simulink model "TxSteering_RxMVDR_4x4_HDL_IQ"  (R2020a)
settings: Solver=FixedStepDiscrete  StartTime=0.0  StopTime=stoptime*0 + inf  RelTol=1e-3
PreLoadFcn:
  | load('iq_bus_obj.mat');
  | model_init
InitFcn:
  | model_init
model workspace (MAT data in the model file):
  socvcb : containers.Map (value not decoded)
values from neighbouring files (symbols this model uses):
  BackSubstitutePrototype = fi(0, matrixdivbacksub_dt)    [model_init.m]
  DataSampleRate = ConverterSampleRate/DecimInterpFactor    (= 245760000)    [model_init.m]
  fc = ConverterSampleRate/4    (= 491520000)    [model_init.m]
  FPGAClkRate = DataSampleRate/VectorSamplingFactor    (= 245760000)    [model_init.m]
  matrixDivDelay = NumberOfCORDICIterations*10 + 86    [model_init.m]
  movavg_bitshift = nextpow2(sqrt(windowSize))    [model_init.m]
  mvdrPipelineDelay = covMatDelay+movAvgDelay+matrixDivDelay+normResponseDelay    [model_init.m]
  NCO_bits = 14    [model_init.m]
  numArrayElements = 4    [model_init.m]
  NumberOfCORDICIterations = matrixdivin_dt.WordLength - 1    [model_init.m]
  S2MM_frame_size = FrameSize*4    (= 40000)    [host_io_init.m]    (also in model_init.m = 1000)
  windowSize = 1024    [model_init.m]
undefined symbols (not defined in the file or in its folder): Fo, Fs, N, physconst
libraries: hdlsllib x268, simulink x53, dspsolvers x1, embreciprocals x1, dsphdlsigops x1
(part 6 of 12)

== system TxSteering_RxMVDR_4x4_HDL_IQ/DUT/MVDR/Compute Weight Vector/Matrix Left Divide/CORDIC/4x4 Complex CORDIC Matrix Left Divide/Q'B, R 4x4 Complex CORDIC Systolic Array/Leading Complex Row Rotation/Rotate first element to real - 1 ==
  x : Inport
  u : Inport  Port=2
  validIn : Inport  Port=3
  Complex to Real-Imag : ComplexToRealImag
  Complex to Real-Imag1 : ComplexToRealImag
  Delay{4..7,9..10,15} (7 alike) : Delay  DelayLength=1
  Force imaginary part to exactly zero : MATLAB Function  TreatAsAtomicUnit=on
  Inverse CORDIC Gain1 : Subsystem  TreatAsAtomicUnit=on  mask{NumberOfCORDICIterations=NumberOfCORDICIterations}
      mask prompts: NumberOfCORDICIterations "Number of CORDIC Iterations"
      mask Display: disp('1/An')
  Inverse CORDIC Gain2 : Subsystem  TreatAsAtomicUnit=on  mask{NumberOfCORDICIterations=NumberOfCORDICIterations}
      mask prompts: NumberOfCORDICIterations "Number of CORDIC Iterations"
      mask Display: disp('1/An')
  Inverse CORDIC Gain3 : Subsystem  TreatAsAtomicUnit=on  mask{NumberOfCORDICIterations=NumberOfCORDICIterations}
      mask prompts: NumberOfCORDICIterations "Number of CORDIC Iterations"
      mask Display: disp('1/An')
  Inverse CORDIC Gain4 : Subsystem  TreatAsAtomicUnit=on  mask{NumberOfCORDICIterations=NumberOfCORDICIterations}
      mask prompts: NumberOfCORDICIterations "Number of CORDIC Iterations"
      mask Display: disp('1/An')
  "Q'B, R Row Rotations - Real" : Subsystem  TreatAsAtomicUnit=on  mask{NumberOfCORDICIterations=NumberOfCORDICIterations}
      mask prompts: NumberOfCORDICIterations "Number of CORDIC Iterations"
  QR 3rd and 4th Quadrant Compensation : MATLAB Function  TreatAsAtomicUnit=on
  Real-Imag to Complex : RealImagToComplex
  Real-Imag to Complex1 : RealImagToComplex
  State Control : StateControl  StateControl=Synchronous
  Unit Delay Enabled Synchronous{,1..3} (4 alike) : hdlsllib/Discrete/Unit Delay Enabled Synchronous  InitialCondition=0.0  SampleTime=-1
      settings: SourceProductBaseCode=SL
  ValidIn to Ready Logic with Delay : Subsystem
  x' : Outport  VectorParamsAs1DForOutWhenUnconnected=off
  u' : Outport  Port=2  VectorParamsAs1DForOutWhenUnconnected=off
  validOut : Outport  Port=3  VectorParamsAs1DForOutWhenUnconnected=off
  ready : Outport  Port=4  VectorParamsAs1DForOutWhenUnconnected=off
  wires:
  Unit Delay Enabled Synchronous3/1 -> x'/1
  Real-Imag to Complex/1 -> Unit Delay Enabled Synchronous3/1
  Unit Delay Enabled Synchronous2/1 -> u'/1
  Real-Imag to Complex1/1 -> Unit Delay Enabled Synchronous2/1
  Unit Delay Enabled Synchronous1/1 -> Complex to Real-Imag/1
  Unit Delay Enabled Synchronous/1 -> Complex to Real-Imag1/1
  "Q'B, R Row Rotations - Real"/6(ready) -> ValidIn to Ready Logic with Delay/1(readyIn)
  ValidIn to Ready Logic with Delay/1(readyOut) -> ready/1
  Delay15/1 -> validOut/1
  "Q'B, R Row Rotations - Real"/5(validOut) -> Delay15/1, Unit Delay Enabled Synchronous3/2, Unit Delay Enabled Synchronous2/2
  Inverse CORDIC Gain3/1(Out1) -> Real-Imag to Complex1/2
  Inverse CORDIC Gain2/1(Out1) -> Real-Imag to Complex1/1
  Inverse CORDIC Gain1/1(Out1) -> Force imaginary part to exactly zero/1(u)
  Inverse CORDIC Gain4/1(Out1) -> Real-Imag to Complex/1
  Delay10/1 -> "Q'B, R Row Rotations - Real"/5(validIn), ValidIn to Ready Logic with Delay/2(validIn * z^-1)
  validIn/1 -> Delay9/1, Unit Delay Enabled Synchronous1/2, Unit Delay Enabled Synchronous/2
  Delay9/1 -> Delay10/1, ValidIn to Ready Logic with Delay/3(validIn)
  Force imaginary part to exactly zero/1(y) -> Real-Imag to Complex/2
  "Q'B, R Row Rotations - Real"/2(y_out) -> Inverse CORDIC Gain1/1(In1)
  u/1 -> Unit Delay Enabled Synchronous/1
  x/1 -> Unit Delay Enabled Synchronous1/1
  "Q'B, R Row Rotations - Real"/4(v_out) -> Inverse CORDIC Gain3/1(In1)
  "Q'B, R Row Rotations - Real"/3(u_out) -> Inverse CORDIC Gain2/1(In1)
  "Q'B, R Row Rotations - Real"/1(x_out) -> Inverse CORDIC Gain4/1(In1)
  Delay7/1 -> "Q'B, R Row Rotations - Real"/4(v)
  Delay6/1 -> "Q'B, R Row Rotations - Real"/3(u)
  Delay5/1 -> "Q'B, R Row Rotations - Real"/2(y)
  Delay4/1 -> "Q'B, R Row Rotations - Real"/1(x)
  Complex to Real-Imag1/2 -> QR 3rd and 4th Quadrant Compensation/4(v)
  Complex to Real-Imag1/1 -> QR 3rd and 4th Quadrant Compensation/3(u)
  Complex to Real-Imag/2 -> QR 3rd and 4th Quadrant Compensation/2(y)
  Complex to Real-Imag/1 -> QR 3rd and 4th Quadrant Compensation/1(x)
  QR 3rd and 4th Quadrant Compensation/4(v_out) -> Delay7/1
  QR 3rd and 4th Quadrant Compensation/2(y_out) -> Delay5/1
  QR 3rd and 4th Quadrant Compensation/3(u_out) -> Delay6/1
  QR 3rd and 4th Quadrant Compensation/1(x_out) -> Delay4/1

== system TxSteering_RxMVDR_4x4_HDL_IQ/DUT/MVDR/Compute Weight Vector/Matrix Left Divide/CORDIC/4x4 Complex CORDIC Matrix Left Divide/Q'B, R 4x4 Complex CORDIC Systolic Array/Leading Complex Row Rotation/ValidIn to Ready Logic ==
  readyIn : Inport
  validIn : Inport  Port=2
  AND : Logic  IconShape=distinctive  AllPortsSameDT=off  OutDataTypeStr=boolean
  NOT : Logic  Operator=NOT  IconShape=distinctive  AllPortsSameDT=off  OutDataTypeStr=boolean
  readyOut : Outport  VectorParamsAs1DForOutWhenUnconnected=off
  wires:
  validIn/1 -> NOT/1
  readyIn/1 -> AND/1
  AND/1 -> readyOut/1
  NOT/1 -> AND/2

== system TxSteering_RxMVDR_4x4_HDL_IQ/DUT/MVDR/Compute Weight Vector/Matrix Left Divide/CORDIC/4x4 Complex CORDIC Matrix Left Divide/Q'B, R 4x4 Complex CORDIC Systolic Array/Leading Complex Row Rotation/ValidIn to Ready Logic1 ==
  readyIn : Inport
  validIn : Inport  Port=2
  AND : Logic  IconShape=distinctive  AllPortsSameDT=off  OutDataTypeStr=boolean
  NOT : Logic  Operator=NOT  IconShape=distinctive  AllPortsSameDT=off  OutDataTypeStr=boolean
  readyOut : Outport  VectorParamsAs1DForOutWhenUnconnected=off
  wires:
  validIn/1 -> NOT/1
  readyIn/1 -> AND/1
  AND/1 -> readyOut/1
  NOT/1 -> AND/2

== system TxSteering_RxMVDR_4x4_HDL_IQ/DUT/MVDR/Compute Weight Vector/Matrix Left Divide/CORDIC/4x4 Complex CORDIC Matrix Left Divide/Q'B, R 4x4 Complex CORDIC Systolic Array/Leading Complex Row Rotation - 2/Inverse CORDIC Gain1 ==
  In1 : Inport
  Inverse CORDIC Gain : Gain  Gain=1/prod(sqrt(1+2.^(-2*(0:double(NumberOfCORDICIterations)-1))))  OutDataTypeStr=Inherit: Same as input
  Out1 : Outport  VectorParamsAs1DForOutWhenUnconnected=off
  wires:
  Inverse CORDIC Gain/1 -> Out1/1
  In1/1 -> Inverse CORDIC Gain/1

== system TxSteering_RxMVDR_4x4_HDL_IQ/DUT/MVDR/Compute Weight Vector/Matrix Left Divide/CORDIC/4x4 Complex CORDIC Matrix Left Divide/Q'B, R 4x4 Complex CORDIC Systolic Array/Leading Complex Row Rotation - 2/Inverse CORDIC Gain2 ==
  In1 : Inport
  Inverse CORDIC Gain : Gain  Gain=1/prod(sqrt(1+2.^(-2*(0:double(NumberOfCORDICIterations)-1))))  OutDataTypeStr=Inherit: Same as input
  Out1 : Outport  VectorParamsAs1DForOutWhenUnconnected=off
  wires:
  Inverse CORDIC Gain/1 -> Out1/1
  In1/1 -> Inverse CORDIC Gain/1

== system TxSteering_RxMVDR_4x4_HDL_IQ/DUT/MVDR/Compute Weight Vector/Matrix Left Divide/CORDIC/4x4 Complex CORDIC Matrix Left Divide/Q'B, R 4x4 Complex CORDIC Systolic Array/Leading Complex Row Rotation - 2/Inverse CORDIC Gain3 ==
  In1 : Inport
  Inverse CORDIC Gain : Gain  Gain=1/prod(sqrt(1+2.^(-2*(0:double(NumberOfCORDICIterations)-1))))  OutDataTypeStr=Inherit: Same as input
  Out1 : Outport  VectorParamsAs1DForOutWhenUnconnected=off
  wires:
  Inverse CORDIC Gain/1 -> Out1/1
  In1/1 -> Inverse CORDIC Gain/1

== system TxSteering_RxMVDR_4x4_HDL_IQ/DUT/MVDR/Compute Weight Vector/Matrix Left Divide/CORDIC/4x4 Complex CORDIC Matrix Left Divide/Q'B, R 4x4 Complex CORDIC Systolic Array/Leading Complex Row Rotation - 2/Inverse CORDIC Gain4 ==
  In1 : Inport
  Inverse CORDIC Gain : Gain  Gain=1/prod(sqrt(1+2.^(-2*(0:double(NumberOfCORDICIterations)-1))))  OutDataTypeStr=Inherit: Same as input
  Out1 : Outport  VectorParamsAs1DForOutWhenUnconnected=off
  wires:
  Inverse CORDIC Gain/1 -> Out1/1
  In1/1 -> Inverse CORDIC Gain/1

== system TxSteering_RxMVDR_4x4_HDL_IQ/DUT/MVDR/Compute Weight Vector/Matrix Left Divide/CORDIC/4x4 Complex CORDIC Matrix Left Divide/Q'B, R 4x4 Complex CORDIC Systolic Array/Leading Complex Row Rotation - 2/Q'B, R Row Rotations - Complex ==
  x : Inport
  y : Inport  Port=2
  u : Inport  Port=3
  v : Inport  Port=4
  validIn : Inport  Port=5
  CORDIC Counter : Subsystem  mask{NumberOfCORDICIterations=NumberOfCORDICIterations}
      mask prompts: NumberOfCORDICIterations "Number of CORDIC Iterations"
  Delay{1..13} (13 alike) : Delay  DelayLength=1
  MATLAB Function : MATLAB Function  TreatAsAtomicUnit=on
  Same Datatype : Subsystem  TreatAsAtomicUnit=on
  Same Datatype1 : Subsystem  TreatAsAtomicUnit=on
  Same Datatype2 : Subsystem  TreatAsAtomicUnit=on
  Same Datatype3 : Subsystem  TreatAsAtomicUnit=on
  Switch{,1..3} (4 alike) : Switch  Criteria=u2 ~= 0
  x_out : Outport  VectorParamsAs1DForOutWhenUnconnected=off
  y_out : Outport  Port=2  VectorParamsAs1DForOutWhenUnconnected=off
  u_out : Outport  Port=3  VectorParamsAs1DForOutWhenUnconnected=off
  v_out : Outport  Port=4  VectorParamsAs1DForOutWhenUnconnected=off
  validOut : Outport  Port=5  VectorParamsAs1DForOutWhenUnconnected=off
  ready : Outport  Port=6  VectorParamsAs1DForOutWhenUnconnected=off
  wires:
  Delay1/1 -> Same Datatype/1(Data), x_out/1
  Delay2/1 -> Same Datatype1/1(Data), y_out/1
  Delay11/1 -> Same Datatype2/1(Data), v_out/1
  MATLAB Function/1(x_out) -> Delay1/1
  MATLAB Function/2(y_out) -> Delay2/1
  MATLAB Function/3(u_out) -> Delay7/1
  MATLAB Function/4(v_out) -> Delay11/1
  Delay7/1 -> Same Datatype3/1(Data), u_out/1
  Delay3/1 -> validOut/1
  validIn/1 -> CORDIC Counter/1(validIn)
  CORDIC Counter/2(count) -> Delay10/1
  CORDIC Counter/3(last) -> Delay12/1
  CORDIC Counter/4(ready) -> Delay13/1
  Switch/1 -> MATLAB Function/1(x)
  Switch1/1 -> MATLAB Function/2(y)
  Switch2/1 -> MATLAB Function/3(u)
  Switch3/1 -> MATLAB Function/4(v)
  CORDIC Counter/1(count_is_positive) -> Delay9/1
  x/1 -> Delay4/1
  y/1 -> Delay5/1
  u/1 -> Delay6/1
  v/1 -> Delay8/1
  Same Datatype/1(DataOut) -> Switch/1
  Same Datatype1/1(DataOut) -> Switch1/1
  Same Datatype3/1(DataOut) -> Switch2/1
  Same Datatype2/1(DataOut) -> Switch3/1
  Delay4/1 -> Same Datatype/2(Reference), Switch/3
  Delay5/1 -> Same Datatype1/2(Reference), Switch1/3
  Delay6/1 -> Same Datatype3/2(Reference), Switch2/3
  Delay8/1 -> Same Datatype2/2(Reference), Switch3/3
  Delay9/1 -> Switch/2, Switch1/2, Switch2/2, Switch3/2
  Delay10/1 -> MATLAB Function/5(iteration)
  Delay12/1 -> Delay3/1
  Delay13/1 -> ready/1

== system TxSteering_RxMVDR_4x4_HDL_IQ/DUT/MVDR/Compute Weight Vector/Matrix Left Divide/CORDIC/4x4 Complex CORDIC Matrix Left Divide/Q'B, R 4x4 Complex CORDIC Systolic Array/Leading Complex Row Rotation - 2/Rotate first element to real ==
  x : Inport
  u : Inport  Port=2
  validIn : Inport  Port=3
  Complex to Real-Imag : ComplexToRealImag
  Complex to Real-Imag1 : ComplexToRealImag
  Delay{4..7,9..10,15} (7 alike) : Delay  DelayLength=1
  Force imaginary part to exactly zero : MATLAB Function  TreatAsAtomicUnit=on
  Inverse CORDIC Gain1 : Subsystem  TreatAsAtomicUnit=on  mask{NumberOfCORDICIterations=NumberOfCORDICIterations}
      mask prompts: NumberOfCORDICIterations "Number of CORDIC Iterations"
      mask Display: disp('1/An')
  Inverse CORDIC Gain2 : Subsystem  TreatAsAtomicUnit=on  mask{NumberOfCORDICIterations=NumberOfCORDICIterations}
      mask prompts: NumberOfCORDICIterations "Number of CORDIC Iterations"
      mask Display: disp('1/An')
  Inverse CORDIC Gain3 : Subsystem  TreatAsAtomicUnit=on  mask{NumberOfCORDICIterations=NumberOfCORDICIterations}
      mask prompts: NumberOfCORDICIterations "Number of CORDIC Iterations"
      mask Display: disp('1/An')
  Inverse CORDIC Gain4 : Subsystem  TreatAsAtomicUnit=on  mask{NumberOfCORDICIterations=NumberOfCORDICIterations}
      mask prompts: NumberOfCORDICIterations "Number of CORDIC Iterations"
      mask Display: disp('1/An')
  "Q'B, R Row Rotations - Real" : Subsystem  TreatAsAtomicUnit=on  mask{NumberOfCORDICIterations=NumberOfCORDICIterations}
      mask prompts: NumberOfCORDICIterations "Number of CORDIC Iterations"
  QR 3rd and 4th Quadrant Compensation : MATLAB Function  TreatAsAtomicUnit=on
  Real-Imag to Complex : RealImagToComplex
  Real-Imag to Complex1 : RealImagToComplex
  State Control : StateControl  StateControl=Synchronous
  Unit Delay Enabled Synchronous{,1..3} (4 alike) : hdlsllib/Discrete/Unit Delay Enabled Synchronous  InitialCondition=0.0  SampleTime=-1
      settings: SourceProductBaseCode=SL
  ValidIn to Ready Logic with Delay : Subsystem
  x' : Outport  VectorParamsAs1DForOutWhenUnconnected=off
  u' : Outport  Port=2  VectorParamsAs1DForOutWhenUnconnected=off
  validOut : Outport  Port=3  VectorParamsAs1DForOutWhenUnconnected=off
  ready : Outport  Port=4  VectorParamsAs1DForOutWhenUnconnected=off
  wires:
  Unit Delay Enabled Synchronous3/1 -> x'/1
  Real-Imag to Complex/1 -> Unit Delay Enabled Synchronous3/1
  Unit Delay Enabled Synchronous2/1 -> u'/1
  Real-Imag to Complex1/1 -> Unit Delay Enabled Synchronous2/1
  Unit Delay Enabled Synchronous1/1 -> Complex to Real-Imag/1
  Unit Delay Enabled Synchronous/1 -> Complex to Real-Imag1/1
  "Q'B, R Row Rotations - Real"/6(ready) -> ValidIn to Ready Logic with Delay/1(readyIn)
  ValidIn to Ready Logic with Delay/1(readyOut) -> ready/1
  Delay15/1 -> validOut/1
  "Q'B, R Row Rotations - Real"/5(validOut) -> Delay15/1, Unit Delay Enabled Synchronous3/2, Unit Delay Enabled Synchronous2/2
  Inverse CORDIC Gain3/1(Out1) -> Real-Imag to Complex1/2
  Inverse CORDIC Gain2/1(Out1) -> Real-Imag to Complex1/1
  Inverse CORDIC Gain1/1(Out1) -> Force imaginary part to exactly zero/1(u)
  Inverse CORDIC Gain4/1(Out1) -> Real-Imag to Complex/1
  Delay10/1 -> "Q'B, R Row Rotations - Real"/5(validIn), ValidIn to Ready Logic with Delay/2(validIn * z^-1)
  validIn/1 -> Delay9/1, Unit Delay Enabled Synchronous1/2, Unit Delay Enabled Synchronous/2
  Delay9/1 -> Delay10/1, ValidIn to Ready Logic with Delay/3(validIn)
  Force imaginary part to exactly zero/1(y) -> Real-Imag to Complex/2
  "Q'B, R Row Rotations - Real"/2(y_out) -> Inverse CORDIC Gain1/1(In1)
  u/1 -> Unit Delay Enabled Synchronous/1
  x/1 -> Unit Delay Enabled Synchronous1/1
  "Q'B, R Row Rotations - Real"/4(v_out) -> Inverse CORDIC Gain3/1(In1)
  "Q'B, R Row Rotations - Real"/3(u_out) -> Inverse CORDIC Gain2/1(In1)
  "Q'B, R Row Rotations - Real"/1(x_out) -> Inverse CORDIC Gain4/1(In1)
  Delay7/1 -> "Q'B, R Row Rotations - Real"/4(v)
  Delay6/1 -> "Q'B, R Row Rotations - Real"/3(u)
  Delay5/1 -> "Q'B, R Row Rotations - Real"/2(y)
  Delay4/1 -> "Q'B, R Row Rotations - Real"/1(x)
  Complex to Real-Imag1/2 -> QR 3rd and 4th Quadrant Compensation/4(v)
  Complex to Real-Imag1/1 -> QR 3rd and 4th Quadrant Compensation/3(u)
  Complex to Real-Imag/2 -> QR 3rd and 4th Quadrant Compensation/2(y)
  Complex to Real-Imag/1 -> QR 3rd and 4th Quadrant Compensation/1(x)
  QR 3rd and 4th Quadrant Compensation/4(v_out) -> Delay7/1
  QR 3rd and 4th Quadrant Compensation/2(y_out) -> Delay5/1
  QR 3rd and 4th Quadrant Compensation/3(u_out) -> Delay6/1
  QR 3rd and 4th Quadrant Compensation/1(x_out) -> Delay4/1

== system TxSteering_RxMVDR_4x4_HDL_IQ/DUT/MVDR/Compute Weight Vector/Matrix Left Divide/CORDIC/4x4 Complex CORDIC Matrix Left Divide/Q'B, R 4x4 Complex CORDIC Systolic Array/Leading Complex Row Rotation - 2/Rotate first element to real - 1 ==
  x : Inport
  u : Inport  Port=2
  validIn : Inport  Port=3
  Complex to Real-Imag : ComplexToRealImag
  Complex to Real-Imag1 : ComplexToRealImag
  Delay{4..7,9..10,15} (7 alike) : Delay  DelayLength=1
  Force imaginary part to exactly zero : MATLAB Function  TreatAsAtomicUnit=on
  Inverse CORDIC Gain1 : Subsystem  TreatAsAtomicUnit=on  mask{NumberOfCORDICIterations=NumberOfCORDICIterations}
      mask prompts: NumberOfCORDICIterations "Number of CORDIC Iterations"
      mask Display: disp('1/An')
  Inverse CORDIC Gain2 : Subsystem  TreatAsAtomicUnit=on  mask{NumberOfCORDICIterations=NumberOfCORDICIterations}
      mask prompts: NumberOfCORDICIterations "Number of CORDIC Iterations"
      mask Display: disp('1/An')
  Inverse CORDIC Gain3 : Subsystem  TreatAsAtomicUnit=on  mask{NumberOfCORDICIterations=NumberOfCORDICIterations}
      mask prompts: NumberOfCORDICIterations "Number of CORDIC Iterations"
      mask Display: disp('1/An')
  Inverse CORDIC Gain4 : Subsystem  TreatAsAtomicUnit=on  mask{NumberOfCORDICIterations=NumberOfCORDICIterations}
      mask prompts: NumberOfCORDICIterations "Number of CORDIC Iterations"
      mask Display: disp('1/An')
  "Q'B, R Row Rotations - Real" : Subsystem  TreatAsAtomicUnit=on  mask{NumberOfCORDICIterations=NumberOfCORDICIterations}
      mask prompts: NumberOfCORDICIterations "Number of CORDIC Iterations"
  QR 3rd and 4th Quadrant Compensation : MATLAB Function  TreatAsAtomicUnit=on
  Real-Imag to Complex : RealImagToComplex
  Real-Imag to Complex1 : RealImagToComplex
  State Control : StateControl  StateControl=Synchronous
  Unit Delay Enabled Synchronous{,1..3} (4 alike) : hdlsllib/Discrete/Unit Delay Enabled Synchronous  InitialCondition=0.0  SampleTime=-1
      settings: SourceProductBaseCode=SL
  ValidIn to Ready Logic with Delay : Subsystem
  x' : Outport  VectorParamsAs1DForOutWhenUnconnected=off
  u' : Outport  Port=2  VectorParamsAs1DForOutWhenUnconnected=off
  validOut : Outport  Port=3  VectorParamsAs1DForOutWhenUnconnected=off
  ready : Outport  Port=4  VectorParamsAs1DForOutWhenUnconnected=off
  wires:
  QR 3rd and 4th Quadrant Compensation/1(x_out) -> Delay4/1
  QR 3rd and 4th Quadrant Compensation/3(u_out) -> Delay6/1
  QR 3rd and 4th Quadrant Compensation/2(y_out) -> Delay5/1
  QR 3rd and 4th Quadrant Compensation/4(v_out) -> Delay7/1
  Complex to Real-Imag/1 -> QR 3rd and 4th Quadrant Compensation/1(x)
  Complex to Real-Imag/2 -> QR 3rd and 4th Quadrant Compensation/2(y)
  Complex to Real-Imag1/1 -> QR 3rd and 4th Quadrant Compensation/3(u)
  Complex to Real-Imag1/2 -> QR 3rd and 4th Quadrant Compensation/4(v)
  Delay4/1 -> "Q'B, R Row Rotations - Real"/1(x)
  Delay5/1 -> "Q'B, R Row Rotations - Real"/2(y)
  Delay6/1 -> "Q'B, R Row Rotations - Real"/3(u)
  Delay7/1 -> "Q'B, R Row Rotations - Real"/4(v)
  "Q'B, R Row Rotations - Real"/1(x_out) -> Inverse CORDIC Gain4/1(In1)
  "Q'B, R Row Rotations - Real"/3(u_out) -> Inverse CORDIC Gain2/1(In1)
  "Q'B, R Row Rotations - Real"/4(v_out) -> Inverse CORDIC Gain3/1(In1)
  x/1 -> Unit Delay Enabled Synchronous1/1
  u/1 -> Unit Delay Enabled Synchronous/1
  "Q'B, R Row Rotations - Real"/2(y_out) -> Inverse CORDIC Gain1/1(In1)
  Force imaginary part to exactly zero/1(y) -> Real-Imag to Complex/2
  Delay9/1 -> ValidIn to Ready Logic with Delay/3(validIn), Delay10/1
  validIn/1 -> Unit Delay Enabled Synchronous/2, Unit Delay Enabled Synchronous1/2, Delay9/1
  Delay10/1 -> ValidIn to Ready Logic with Delay/2(validIn * z^-1), "Q'B, R Row Rotations - Real"/5(validIn)
  Inverse CORDIC Gain4/1(Out1) -> Real-Imag to Complex/1
  Inverse CORDIC Gain1/1(Out1) -> Force imaginary part to exactly zero/1(u)
  Inverse CORDIC Gain2/1(Out1) -> Real-Imag to Complex1/1
  Inverse CORDIC Gain3/1(Out1) -> Real-Imag to Complex1/2
  "Q'B, R Row Rotations - Real"/5(validOut) -> Unit Delay Enabled Synchronous2/2, Unit Delay Enabled Synchronous3/2, Delay15/1
  Delay15/1 -> validOut/1
  ValidIn to Ready Logic with Delay/1(readyOut) -> ready/1
  "Q'B, R Row Rotations - Real"/6(ready) -> ValidIn to Ready Logic with Delay/1(readyIn)
  Unit Delay Enabled Synchronous/1 -> Complex to Real-Imag1/1
  Unit Delay Enabled Synchronous1/1 -> Complex to Real-Imag/1
  Real-Imag to Complex1/1 -> Unit Delay Enabled Synchronous2/1
  Unit Delay Enabled Synchronous2/1 -> u'/1
  Real-Imag to Complex/1 -> Unit Delay Enabled Synchronous3/1
  Unit Delay Enabled Synchronous3/1 -> x'/1

== system TxSteering_RxMVDR_4x4_HDL_IQ/DUT/MVDR/Compute Weight Vector/Matrix Left Divide/CORDIC/4x4 Complex CORDIC Matrix Left Divide/Q'B, R 4x4 Complex CORDIC Systolic Array/Leading Complex Row Rotation - 2/ValidIn to Ready Logic ==
  readyIn : Inport
  validIn : Inport  Port=2
  AND : Logic  IconShape=distinctive  AllPortsSameDT=off  OutDataTypeStr=boolean
  NOT : Logic  Operator=NOT  IconShape=distinctive  AllPortsSameDT=off  OutDataTypeStr=boolean
  readyOut : Outport  VectorParamsAs1DForOutWhenUnconnected=off
  wires:
  validIn/1 -> NOT/1
  readyIn/1 -> AND/1
  AND/1 -> readyOut/1
  NOT/1 -> AND/2

== system TxSteering_RxMVDR_4x4_HDL_IQ/DUT/MVDR/Compute Weight Vector/Matrix Left Divide/CORDIC/4x4 Complex CORDIC Matrix Left Divide/Q'B, R 4x4 Complex CORDIC Systolic Array/Leading Complex Row Rotation - 2/ValidIn to Ready Logic1 ==
  readyIn : Inport
  validIn : Inport  Port=2
  AND : Logic  IconShape=distinctive  AllPortsSameDT=off  OutDataTypeStr=boolean
  NOT : Logic  Operator=NOT  IconShape=distinctive  AllPortsSameDT=off  OutDataTypeStr=boolean
  readyOut : Outport  VectorParamsAs1DForOutWhenUnconnected=off
  wires:
  validIn/1 -> NOT/1
  readyIn/1 -> AND/1
  AND/1 -> readyOut/1
  NOT/1 -> AND/2

== system TxSteering_RxMVDR_4x4_HDL_IQ/DUT/MVDR/Compute Weight Vector/Matrix Left Divide/CORDIC/4x4 Complex CORDIC Matrix Left Divide/Q'B, R 4x4 Complex CORDIC Systolic Array/Leading Complex Row Rotation - 3/Inverse CORDIC Gain1 ==
  In1 : Inport
  Inverse CORDIC Gain : Gain  Gain=1/prod(sqrt(1+2.^(-2*(0:double(NumberOfCORDICIterations)-1))))  OutDataTypeStr=Inherit: Same as input
  Out1 : Outport  VectorParamsAs1DForOutWhenUnconnected=off
  wires:
  Inverse CORDIC Gain/1 -> Out1/1
  In1/1 -> Inverse CORDIC Gain/1

== system TxSteering_RxMVDR_4x4_HDL_IQ/DUT/MVDR/Compute Weight Vector/Matrix Left Divide/CORDIC/4x4 Complex CORDIC Matrix Left Divide/Q'B, R 4x4 Complex CORDIC Systolic Array/Leading Complex Row Rotation - 3/Inverse CORDIC Gain2 ==
  In1 : Inport
  Inverse CORDIC Gain : Gain  Gain=1/prod(sqrt(1+2.^(-2*(0:double(NumberOfCORDICIterations)-1))))  OutDataTypeStr=Inherit: Same as input
  Out1 : Outport  VectorParamsAs1DForOutWhenUnconnected=off
  wires:
  Inverse CORDIC Gain/1 -> Out1/1
  In1/1 -> Inverse CORDIC Gain/1

== system TxSteering_RxMVDR_4x4_HDL_IQ/DUT/MVDR/Compute Weight Vector/Matrix Left Divide/CORDIC/4x4 Complex CORDIC Matrix Left Divide/Q'B, R 4x4 Complex CORDIC Systolic Array/Leading Complex Row Rotation - 3/Inverse CORDIC Gain3 ==
  In1 : Inport
  Inverse CORDIC Gain : Gain  Gain=1/prod(sqrt(1+2.^(-2*(0:double(NumberOfCORDICIterations)-1))))  OutDataTypeStr=Inherit: Same as input
  Out1 : Outport  VectorParamsAs1DForOutWhenUnconnected=off
  wires:
  Inverse CORDIC Gain/1 -> Out1/1
  In1/1 -> Inverse CORDIC Gain/1

== system TxSteering_RxMVDR_4x4_HDL_IQ/DUT/MVDR/Compute Weight Vector/Matrix Left Divide/CORDIC/4x4 Complex CORDIC Matrix Left Divide/Q'B, R 4x4 Complex CORDIC Systolic Array/Leading Complex Row Rotation - 3/Inverse CORDIC Gain4 ==
  In1 : Inport
  Inverse CORDIC Gain : Gain  Gain=1/prod(sqrt(1+2.^(-2*(0:double(NumberOfCORDICIterations)-1))))  OutDataTypeStr=Inherit: Same as input
  Out1 : Outport  VectorParamsAs1DForOutWhenUnconnected=off
  wires:
  Inverse CORDIC Gain/1 -> Out1/1
  In1/1 -> Inverse CORDIC Gain/1

== system TxSteering_RxMVDR_4x4_HDL_IQ/DUT/MVDR/Compute Weight Vector/Matrix Left Divide/CORDIC/4x4 Complex CORDIC Matrix Left Divide/Q'B, R 4x4 Complex CORDIC Systolic Array/Leading Complex Row Rotation - 3/Q'B, R Row Rotations - Complex ==
  x : Inport
  y : Inport  Port=2
  u : Inport  Port=3
  v : Inport  Port=4
  validIn : Inport  Port=5
  CORDIC Counter : Subsystem  mask{NumberOfCORDICIterations=NumberOfCORDICIterations}
      mask prompts: NumberOfCORDICIterations "Number of CORDIC Iterations"
  Delay{1..13} (13 alike) : Delay  DelayLength=1
  MATLAB Function : MATLAB Function  TreatAsAtomicUnit=on
  Same Datatype : Subsystem  TreatAsAtomicUnit=on
  Same Datatype1 : Subsystem  TreatAsAtomicUnit=on
  Same Datatype2 : Subsystem  TreatAsAtomicUnit=on
  Same Datatype3 : Subsystem  TreatAsAtomicUnit=on
  Switch{,1..3} (4 alike) : Switch  Criteria=u2 ~= 0
  x_out : Outport  VectorParamsAs1DForOutWhenUnconnected=off
  y_out : Outport  Port=2  VectorParamsAs1DForOutWhenUnconnected=off
  u_out : Outport  Port=3  VectorParamsAs1DForOutWhenUnconnected=off
  v_out : Outport  Port=4  VectorParamsAs1DForOutWhenUnconnected=off
  validOut : Outport  Port=5  VectorParamsAs1DForOutWhenUnconnected=off
  ready : Outport  Port=6  VectorParamsAs1DForOutWhenUnconnected=off
  wires:
  Delay13/1 -> ready/1
  Delay12/1 -> Delay3/1
  Delay10/1 -> MATLAB Function/5(iteration)
  Delay9/1 -> Switch3/2, Switch2/2, Switch1/2, Switch/2
  Delay8/1 -> Switch3/3, Same Datatype2/2(Reference)
  Delay6/1 -> Switch2/3, Same Datatype3/2(Reference)
  Delay5/1 -> Switch1/3, Same Datatype1/2(Reference)
  Delay4/1 -> Switch/3, Same Datatype/2(Reference)
  Same Datatype2/1(DataOut) -> Switch3/1
  Same Datatype3/1(DataOut) -> Switch2/1
  Same Datatype1/1(DataOut) -> Switch1/1
  Same Datatype/1(DataOut) -> Switch/1
  v/1 -> Delay8/1
  u/1 -> Delay6/1
  y/1 -> Delay5/1
  x/1 -> Delay4/1
  CORDIC Counter/1(count_is_positive) -> Delay9/1
  Switch3/1 -> MATLAB Function/4(v)
  Switch2/1 -> MATLAB Function/3(u)
  Switch1/1 -> MATLAB Function/2(y)
  Switch/1 -> MATLAB Function/1(x)
  CORDIC Counter/4(ready) -> Delay13/1
  CORDIC Counter/3(last) -> Delay12/1
  CORDIC Counter/2(count) -> Delay10/1
  validIn/1 -> CORDIC Counter/1(validIn)
  Delay3/1 -> validOut/1
  Delay7/1 -> u_out/1, Same Datatype3/1(Data)
  MATLAB Function/4(v_out) -> Delay11/1
  MATLAB Function/3(u_out) -> Delay7/1
  MATLAB Function/2(y_out) -> Delay2/1
  MATLAB Function/1(x_out) -> Delay1/1
  Delay11/1 -> v_out/1, Same Datatype2/1(Data)
  Delay2/1 -> y_out/1, Same Datatype1/1(Data)
  Delay1/1 -> x_out/1, Same Datatype/1(Data)

== system TxSteering_RxMVDR_4x4_HDL_IQ/DUT/MVDR/Compute Weight Vector/Matrix Left Divide/CORDIC/4x4 Complex CORDIC Matrix Left Divide/Q'B, R 4x4 Complex CORDIC Systolic Array/Leading Complex Row Rotation - 3/Rotate first element to real ==
  x : Inport
  u : Inport  Port=2
  validIn : Inport  Port=3
  Complex to Real-Imag : ComplexToRealImag
  Complex to Real-Imag1 : ComplexToRealImag
  Delay{4..7,9..10,15} (7 alike) : Delay  DelayLength=1
  Force imaginary part to exactly zero : MATLAB Function  TreatAsAtomicUnit=on
  Inverse CORDIC Gain1 : Subsystem  TreatAsAtomicUnit=on  mask{NumberOfCORDICIterations=NumberOfCORDICIterations}
      mask prompts: NumberOfCORDICIterations "Number of CORDIC Iterations"
      mask Display: disp('1/An')
  Inverse CORDIC Gain2 : Subsystem  TreatAsAtomicUnit=on  mask{NumberOfCORDICIterations=NumberOfCORDICIterations}
      mask prompts: NumberOfCORDICIterations "Number of CORDIC Iterations"
      mask Display: disp('1/An')
  Inverse CORDIC Gain3 : Subsystem  TreatAsAtomicUnit=on  mask{NumberOfCORDICIterations=NumberOfCORDICIterations}
      mask prompts: NumberOfCORDICIterations "Number of CORDIC Iterations"
      mask Display: disp('1/An')
  Inverse CORDIC Gain4 : Subsystem  TreatAsAtomicUnit=on  mask{NumberOfCORDICIterations=NumberOfCORDICIterations}
      mask prompts: NumberOfCORDICIterations "Number of CORDIC Iterations"
      mask Display: disp('1/An')
  "Q'B, R Row Rotations - Real" : Subsystem  TreatAsAtomicUnit=on  mask{NumberOfCORDICIterations=NumberOfCORDICIterations}
      mask prompts: NumberOfCORDICIterations "Number of CORDIC Iterations"
  QR 3rd and 4th Quadrant Compensation : MATLAB Function  TreatAsAtomicUnit=on
  Real-Imag to Complex : RealImagToComplex
  Real-Imag to Complex1 : RealImagToComplex
  State Control : StateControl  StateControl=Synchronous
  Unit Delay Enabled Synchronous{,1..3} (4 alike) : hdlsllib/Discrete/Unit Delay Enabled Synchronous  InitialCondition=0.0  SampleTime=-1
      settings: SourceProductBaseCode=SL
  ValidIn to Ready Logic with Delay : Subsystem
  x' : Outport  VectorParamsAs1DForOutWhenUnconnected=off
  u' : Outport  Port=2  VectorParamsAs1DForOutWhenUnconnected=off
  validOut : Outport  Port=3  VectorParamsAs1DForOutWhenUnconnected=off
  ready : Outport  Port=4  VectorParamsAs1DForOutWhenUnconnected=off
  wires:
  Unit Delay Enabled Synchronous3/1 -> x'/1
  Real-Imag to Complex/1 -> Unit Delay Enabled Synchronous3/1
  Unit Delay Enabled Synchronous2/1 -> u'/1
  Real-Imag to Complex1/1 -> Unit Delay Enabled Synchronous2/1
  Unit Delay Enabled Synchronous1/1 -> Complex to Real-Imag/1
  Unit Delay Enabled Synchronous/1 -> Complex to Real-Imag1/1
  "Q'B, R Row Rotations - Real"/6(ready) -> ValidIn to Ready Logic with Delay/1(readyIn)
  ValidIn to Ready Logic with Delay/1(readyOut) -> ready/1
  Delay15/1 -> validOut/1
  "Q'B, R Row Rotations - Real"/5(validOut) -> Delay15/1, Unit Delay Enabled Synchronous3/2, Unit Delay Enabled Synchronous2/2
  Inverse CORDIC Gain3/1(Out1) -> Real-Imag to Complex1/2
  Inverse CORDIC Gain2/1(Out1) -> Real-Imag to Complex1/1
  Inverse CORDIC Gain1/1(Out1) -> Force imaginary part to exactly zero/1(u)
  Inverse CORDIC Gain4/1(Out1) -> Real-Imag to Complex/1
  Delay10/1 -> "Q'B, R Row Rotations - Real"/5(validIn), ValidIn to Ready Logic with Delay/2(validIn * z^-1)
  validIn/1 -> Delay9/1, Unit Delay Enabled Synchronous1/2, Unit Delay Enabled Synchronous/2
  Delay9/1 -> Delay10/1, ValidIn to Ready Logic with Delay/3(validIn)
  Force imaginary part to exactly zero/1(y) -> Real-Imag to Complex/2
  "Q'B, R Row Rotations - Real"/2(y_out) -> Inverse CORDIC Gain1/1(In1)
  u/1 -> Unit Delay Enabled Synchronous/1
  x/1 -> Unit Delay Enabled Synchronous1/1
  "Q'B, R Row Rotations - Real"/4(v_out) -> Inverse CORDIC Gain3/1(In1)
  "Q'B, R Row Rotations - Real"/3(u_out) -> Inverse CORDIC Gain2/1(In1)
  "Q'B, R Row Rotations - Real"/1(x_out) -> Inverse CORDIC Gain4/1(In1)
  Delay7/1 -> "Q'B, R Row Rotations - Real"/4(v)
  Delay6/1 -> "Q'B, R Row Rotations - Real"/3(u)
  Delay5/1 -> "Q'B, R Row Rotations - Real"/2(y)
  Delay4/1 -> "Q'B, R Row Rotations - Real"/1(x)
  Complex to Real-Imag1/2 -> QR 3rd and 4th Quadrant Compensation/4(v)
  Complex to Real-Imag1/1 -> QR 3rd and 4th Quadrant Compensation/3(u)
  Complex to Real-Imag/2 -> QR 3rd and 4th Quadrant Compensation/2(y)
  Complex to Real-Imag/1 -> QR 3rd and 4th Quadrant Compensation/1(x)
  QR 3rd and 4th Quadrant Compensation/4(v_out) -> Delay7/1
  QR 3rd and 4th Quadrant Compensation/2(y_out) -> Delay5/1
  QR 3rd and 4th Quadrant Compensation/3(u_out) -> Delay6/1
  QR 3rd and 4th Quadrant Compensation/1(x_out) -> Delay4/1

== system TxSteering_RxMVDR_4x4_HDL_IQ/DUT/MVDR/Compute Weight Vector/Matrix Left Divide/CORDIC/4x4 Complex CORDIC Matrix Left Divide/Q'B, R 4x4 Complex CORDIC Systolic Array/Leading Complex Row Rotation - 3/Rotate first element to real - 1 ==
  x : Inport
  u : Inport  Port=2
  validIn : Inport  Port=3
  Complex to Real-Imag : ComplexToRealImag
  Complex to Real-Imag1 : ComplexToRealImag
  Delay{4..7,9..10,15} (7 alike) : Delay  DelayLength=1
  Force imaginary part to exactly zero : MATLAB Function  TreatAsAtomicUnit=on
  Inverse CORDIC Gain1 : Subsystem  TreatAsAtomicUnit=on  mask{NumberOfCORDICIterations=NumberOfCORDICIterations}
      mask prompts: NumberOfCORDICIterations "Number of CORDIC Iterations"
      mask Display: disp('1/An')
  Inverse CORDIC Gain2 : Subsystem  TreatAsAtomicUnit=on  mask{NumberOfCORDICIterations=NumberOfCORDICIterations}
      mask prompts: NumberOfCORDICIterations "Number of CORDIC Iterations"
      mask Display: disp('1/An')
  Inverse CORDIC Gain3 : Subsystem  TreatAsAtomicUnit=on  mask{NumberOfCORDICIterations=NumberOfCORDICIterations}
      mask prompts: NumberOfCORDICIterations "Number of CORDIC Iterations"
      mask Display: disp('1/An')
  Inverse CORDIC Gain4 : Subsystem  TreatAsAtomicUnit=on  mask{NumberOfCORDICIterations=NumberOfCORDICIterations}
      mask prompts: NumberOfCORDICIterations "Number of CORDIC Iterations"
      mask Display: disp('1/An')
  "Q'B, R Row Rotations - Real" : Subsystem  TreatAsAtomicUnit=on  mask{NumberOfCORDICIterations=NumberOfCORDICIterations}
      mask prompts: NumberOfCORDICIterations "Number of CORDIC Iterations"
  QR 3rd and 4th Quadrant Compensation : MATLAB Function  TreatAsAtomicUnit=on
  Real-Imag to Complex : RealImagToComplex
  Real-Imag to Complex1 : RealImagToComplex
  State Control : StateControl  StateControl=Synchronous
  Unit Delay Enabled Synchronous{,1..3} (4 alike) : hdlsllib/Discrete/Unit Delay Enabled Synchronous  InitialCondition=0.0  SampleTime=-1
      settings: SourceProductBaseCode=SL
  ValidIn to Ready Logic with Delay : Subsystem
  x' : Outport  VectorParamsAs1DForOutWhenUnconnected=off
  u' : Outport  Port=2  VectorParamsAs1DForOutWhenUnconnected=off
  validOut : Outport  Port=3  VectorParamsAs1DForOutWhenUnconnected=off
  ready : Outport  Port=4  VectorParamsAs1DForOutWhenUnconnected=off
  wires:
  Unit Delay Enabled Synchronous3/1 -> x'/1
  Real-Imag to Complex/1 -> Unit Delay Enabled Synchronous3/1
  Unit Delay Enabled Synchronous2/1 -> u'/1
  Real-Imag to Complex1/1 -> Unit Delay Enabled Synchronous2/1
  Unit Delay Enabled Synchronous1/1 -> Complex to Real-Imag/1
  Unit Delay Enabled Synchronous/1 -> Complex to Real-Imag1/1
  "Q'B, R Row Rotations - Real"/6(ready) -> ValidIn to Ready Logic with Delay/1(readyIn)
  ValidIn to Ready Logic with Delay/1(readyOut) -> ready/1
  Delay15/1 -> validOut/1
  "Q'B, R Row Rotations - Real"/5(validOut) -> Delay15/1, Unit Delay Enabled Synchronous3/2, Unit Delay Enabled Synchronous2/2
  Inverse CORDIC Gain3/1(Out1) -> Real-Imag to Complex1/2
  Inverse CORDIC Gain2/1(Out1) -> Real-Imag to Complex1/1
  Inverse CORDIC Gain1/1(Out1) -> Force imaginary part to exactly zero/1(u)
  Inverse CORDIC Gain4/1(Out1) -> Real-Imag to Complex/1
  Delay10/1 -> "Q'B, R Row Rotations - Real"/5(validIn), ValidIn to Ready Logic with Delay/2(validIn * z^-1)
  validIn/1 -> Delay9/1, Unit Delay Enabled Synchronous1/2, Unit Delay Enabled Synchronous/2
  Delay9/1 -> Delay10/1, ValidIn to Ready Logic with Delay/3(validIn)
  Force imaginary part to exactly zero/1(y) -> Real-Imag to Complex/2
  "Q'B, R Row Rotations - Real"/2(y_out) -> Inverse CORDIC Gain1/1(In1)
  u/1 -> Unit Delay Enabled Synchronous/1
  x/1 -> Unit Delay Enabled Synchronous1/1
  "Q'B, R Row Rotations - Real"/4(v_out) -> Inverse CORDIC Gain3/1(In1)
  "Q'B, R Row Rotations - Real"/3(u_out) -> Inverse CORDIC Gain2/1(In1)
  "Q'B, R Row Rotations - Real"/1(x_out) -> Inverse CORDIC Gain4/1(In1)
  Delay7/1 -> "Q'B, R Row Rotations - Real"/4(v)
  Delay6/1 -> "Q'B, R Row Rotations - Real"/3(u)
  Delay5/1 -> "Q'B, R Row Rotations - Real"/2(y)
  Delay4/1 -> "Q'B, R Row Rotations - Real"/1(x)
  Complex to Real-Imag1/2 -> QR 3rd and 4th Quadrant Compensation/4(v)
  Complex to Real-Imag1/1 -> QR 3rd and 4th Quadrant Compensation/3(u)
  Complex to Real-Imag/2 -> QR 3rd and 4th Quadrant Compensation/2(y)
  Complex to Real-Imag/1 -> QR 3rd and 4th Quadrant Compensation/1(x)
  QR 3rd and 4th Quadrant Compensation/4(v_out) -> Delay7/1
  QR 3rd and 4th Quadrant Compensation/2(y_out) -> Delay5/1
  QR 3rd and 4th Quadrant Compensation/3(u_out) -> Delay6/1
  QR 3rd and 4th Quadrant Compensation/1(x_out) -> Delay4/1

== system TxSteering_RxMVDR_4x4_HDL_IQ/DUT/MVDR/Compute Weight Vector/Matrix Left Divide/CORDIC/4x4 Complex CORDIC Matrix Left Divide/Q'B, R 4x4 Complex CORDIC Systolic Array/Leading Complex Row Rotation - 3/ValidIn to Ready Logic ==
  readyIn : Inport
  validIn : Inport  Port=2
  AND : Logic  IconShape=distinctive  AllPortsSameDT=off  OutDataTypeStr=boolean
  NOT : Logic  Operator=NOT  IconShape=distinctive  AllPortsSameDT=off  OutDataTypeStr=boolean
  readyOut : Outport  VectorParamsAs1DForOutWhenUnconnected=off
  wires:
  validIn/1 -> NOT/1
  readyIn/1 -> AND/1
  AND/1 -> readyOut/1
  NOT/1 -> AND/2

== system TxSteering_RxMVDR_4x4_HDL_IQ/DUT/MVDR/Compute Weight Vector/Matrix Left Divide/CORDIC/4x4 Complex CORDIC Matrix Left Divide/Q'B, R 4x4 Complex CORDIC Systolic Array/Leading Complex Row Rotation - 3/ValidIn to Ready Logic1 ==
  readyIn : Inport
  validIn : Inport  Port=2
  AND : Logic  IconShape=distinctive  AllPortsSameDT=off  OutDataTypeStr=boolean
  NOT : Logic  Operator=NOT  IconShape=distinctive  AllPortsSameDT=off  OutDataTypeStr=boolean
  readyOut : Outport  VectorParamsAs1DForOutWhenUnconnected=off
  wires:
  validIn/1 -> NOT/1
  readyIn/1 -> AND/1
  AND/1 -> readyOut/1
  NOT/1 -> AND/2

== system TxSteering_RxMVDR_4x4_HDL_IQ/DUT/MVDR/Compute Weight Vector/Matrix Left Divide/CORDIC/4x4 Complex CORDIC Matrix Left Divide/Q'B, R 4x4 Complex CORDIC Systolic Array/Leading Complex Row Rotation - 4/Inverse CORDIC Gain1 ==
  In1 : Inport
  Inverse CORDIC Gain : Gain  Gain=1/prod(sqrt(1+2.^(-2*(0:double(NumberOfCORDICIterations)-1))))  OutDataTypeStr=Inherit: Same as input
  Out1 : Outport  VectorParamsAs1DForOutWhenUnconnected=off
  wires:
  Inverse CORDIC Gain/1 -> Out1/1
  In1/1 -> Inverse CORDIC Gain/1

== system TxSteering_RxMVDR_4x4_HDL_IQ/DUT/MVDR/Compute Weight Vector/Matrix Left Divide/CORDIC/4x4 Complex CORDIC Matrix Left Divide/Q'B, R 4x4 Complex CORDIC Systolic Array/Leading Complex Row Rotation - 4/Inverse CORDIC Gain2 ==
  In1 : Inport
  Inverse CORDIC Gain : Gain  Gain=1/prod(sqrt(1+2.^(-2*(0:double(NumberOfCORDICIterations)-1))))  OutDataTypeStr=Inherit: Same as input
  Out1 : Outport  VectorParamsAs1DForOutWhenUnconnected=off
  wires:
  Inverse CORDIC Gain/1 -> Out1/1
  In1/1 -> Inverse CORDIC Gain/1

== system TxSteering_RxMVDR_4x4_HDL_IQ/DUT/MVDR/Compute Weight Vector/Matrix Left Divide/CORDIC/4x4 Complex CORDIC Matrix Left Divide/Q'B, R 4x4 Complex CORDIC Systolic Array/Leading Complex Row Rotation - 4/Inverse CORDIC Gain3 ==
  In1 : Inport
  Inverse CORDIC Gain : Gain  Gain=1/prod(sqrt(1+2.^(-2*(0:double(NumberOfCORDICIterations)-1))))  OutDataTypeStr=Inherit: Same as input
  Out1 : Outport  VectorParamsAs1DForOutWhenUnconnected=off
  wires:
  Inverse CORDIC Gain/1 -> Out1/1
  In1/1 -> Inverse CORDIC Gain/1

== system TxSteering_RxMVDR_4x4_HDL_IQ/DUT/MVDR/Compute Weight Vector/Matrix Left Divide/CORDIC/4x4 Complex CORDIC Matrix Left Divide/Q'B, R 4x4 Complex CORDIC Systolic Array/Leading Complex Row Rotation - 4/Inverse CORDIC Gain4 ==
  In1 : Inport
  Inverse CORDIC Gain : Gain  Gain=1/prod(sqrt(1+2.^(-2*(0:double(NumberOfCORDICIterations)-1))))  OutDataTypeStr=Inherit: Same as input
  Out1 : Outport  VectorParamsAs1DForOutWhenUnconnected=off
  wires:
  Inverse CORDIC Gain/1 -> Out1/1
  In1/1 -> Inverse CORDIC Gain/1

== system TxSteering_RxMVDR_4x4_HDL_IQ/DUT/MVDR/Compute Weight Vector/Matrix Left Divide/CORDIC/4x4 Complex CORDIC Matrix Left Divide/Q'B, R 4x4 Complex CORDIC Systolic Array/Leading Complex Row Rotation - 4/Q'B, R Row Rotations - Complex ==
  x : Inport
  y : Inport  Port=2
  u : Inport  Port=3
  v : Inport  Port=4
  validIn : Inport  Port=5
  CORDIC Counter : Subsystem  mask{NumberOfCORDICIterations=NumberOfCORDICIterations}
      mask prompts: NumberOfCORDICIterations "Number of CORDIC Iterations"
  Delay{1..13} (13 alike) : Delay  DelayLength=1
  MATLAB Function : MATLAB Function  TreatAsAtomicUnit=on
  Same Datatype : Subsystem  TreatAsAtomicUnit=on
  Same Datatype1 : Subsystem  TreatAsAtomicUnit=on
  Same Datatype2 : Subsystem  TreatAsAtomicUnit=on
  Same Datatype3 : Subsystem  TreatAsAtomicUnit=on
  Switch{,1..3} (4 alike) : Switch  Criteria=u2 ~= 0
  x_out : Outport  VectorParamsAs1DForOutWhenUnconnected=off
  y_out : Outport  Port=2  VectorParamsAs1DForOutWhenUnconnected=off
  u_out : Outport  Port=3  VectorParamsAs1DForOutWhenUnconnected=off
  v_out : Outport  Port=4  VectorParamsAs1DForOutWhenUnconnected=off
  validOut : Outport  Port=5  VectorParamsAs1DForOutWhenUnconnected=off
  ready : Outport  Port=6  VectorParamsAs1DForOutWhenUnconnected=off
  wires:
  Delay13/1 -> ready/1
  Delay12/1 -> Delay3/1
  Delay10/1 -> MATLAB Function/5(iteration)
  Delay9/1 -> Switch3/2, Switch2/2, Switch1/2, Switch/2
  Delay8/1 -> Switch3/3, Same Datatype2/2(Reference)
  Delay6/1 -> Switch2/3, Same Datatype3/2(Reference)
  Delay5/1 -> Switch1/3, Same Datatype1/2(Reference)
  Delay4/1 -> Switch/3, Same Datatype/2(Reference)
  Same Datatype2/1(DataOut) -> Switch3/1
  Same Datatype3/1(DataOut) -> Switch2/1
  Same Datatype1/1(DataOut) -> Switch1/1
  Same Datatype/1(DataOut) -> Switch/1
  v/1 -> Delay8/1
  u/1 -> Delay6/1
  y/1 -> Delay5/1
  x/1 -> Delay4/1
  CORDIC Counter/1(count_is_positive) -> Delay9/1
  Switch3/1 -> MATLAB Function/4(v)
  Switch2/1 -> MATLAB Function/3(u)
  Switch1/1 -> MATLAB Function/2(y)
  Switch/1 -> MATLAB Function/1(x)
  CORDIC Counter/4(ready) -> Delay13/1
  CORDIC Counter/3(last) -> Delay12/1
  CORDIC Counter/2(count) -> Delay10/1
  validIn/1 -> CORDIC Counter/1(validIn)
  Delay3/1 -> validOut/1
  Delay7/1 -> u_out/1, Same Datatype3/1(Data)
  MATLAB Function/4(v_out) -> Delay11/1
  MATLAB Function/3(u_out) -> Delay7/1
  MATLAB Function/2(y_out) -> Delay2/1
  MATLAB Function/1(x_out) -> Delay1/1
  Delay11/1 -> v_out/1, Same Datatype2/1(Data)
  Delay2/1 -> y_out/1, Same Datatype1/1(Data)
  Delay1/1 -> x_out/1, Same Datatype/1(Data)

== system TxSteering_RxMVDR_4x4_HDL_IQ/DUT/MVDR/Compute Weight Vector/Matrix Left Divide/CORDIC/4x4 Complex CORDIC Matrix Left Divide/Q'B, R 4x4 Complex CORDIC Systolic Array/Leading Complex Row Rotation - 4/Rotate first element to real ==
  x : Inport
  u : Inport  Port=2
  validIn : Inport  Port=3
  Complex to Real-Imag : ComplexToRealImag
  Complex to Real-Imag1 : ComplexToRealImag
  Delay{4..7,9..10,15} (7 alike) : Delay  DelayLength=1
  Force imaginary part to exactly zero : MATLAB Function  TreatAsAtomicUnit=on
  Inverse CORDIC Gain1 : Subsystem  TreatAsAtomicUnit=on  mask{NumberOfCORDICIterations=NumberOfCORDICIterations}
      mask prompts: NumberOfCORDICIterations "Number of CORDIC Iterations"
      mask Display: disp('1/An')
  Inverse CORDIC Gain2 : Subsystem  TreatAsAtomicUnit=on  mask{NumberOfCORDICIterations=NumberOfCORDICIterations}
      mask prompts: NumberOfCORDICIterations "Number of CORDIC Iterations"
      mask Display: disp('1/An')
  Inverse CORDIC Gain3 : Subsystem  TreatAsAtomicUnit=on  mask{NumberOfCORDICIterations=NumberOfCORDICIterations}
      mask prompts: NumberOfCORDICIterations "Number of CORDIC Iterations"
      mask Display: disp('1/An')
  Inverse CORDIC Gain4 : Subsystem  TreatAsAtomicUnit=on  mask{NumberOfCORDICIterations=NumberOfCORDICIterations}
      mask prompts: NumberOfCORDICIterations "Number of CORDIC Iterations"
      mask Display: disp('1/An')
  "Q'B, R Row Rotations - Real" : Subsystem  TreatAsAtomicUnit=on  mask{NumberOfCORDICIterations=NumberOfCORDICIterations}
      mask prompts: NumberOfCORDICIterations "Number of CORDIC Iterations"
  QR 3rd and 4th Quadrant Compensation : MATLAB Function  TreatAsAtomicUnit=on
  Real-Imag to Complex : RealImagToComplex
  Real-Imag to Complex1 : RealImagToComplex
  State Control : StateControl  StateControl=Synchronous
  Unit Delay Enabled Synchronous{,1..3} (4 alike) : hdlsllib/Discrete/Unit Delay Enabled Synchronous  InitialCondition=0.0  SampleTime=-1
      settings: SourceProductBaseCode=SL
  ValidIn to Ready Logic with Delay : Subsystem
  x' : Outport  VectorParamsAs1DForOutWhenUnconnected=off
  u' : Outport  Port=2  VectorParamsAs1DForOutWhenUnconnected=off
  validOut : Outport  Port=3  VectorParamsAs1DForOutWhenUnconnected=off
  ready : Outport  Port=4  VectorParamsAs1DForOutWhenUnconnected=off
  wires:
  QR 3rd and 4th Quadrant Compensation/1(x_out) -> Delay4/1
  QR 3rd and 4th Quadrant Compensation/3(u_out) -> Delay6/1
  QR 3rd and 4th Quadrant Compensation/2(y_out) -> Delay5/1
  QR 3rd and 4th Quadrant Compensation/4(v_out) -> Delay7/1
  Complex to Real-Imag/1 -> QR 3rd and 4th Quadrant Compensation/1(x)
  Complex to Real-Imag/2 -> QR 3rd and 4th Quadrant Compensation/2(y)
  Complex to Real-Imag1/1 -> QR 3rd and 4th Quadrant Compensation/3(u)
  Complex to Real-Imag1/2 -> QR 3rd and 4th Quadrant Compensation/4(v)
  Delay4/1 -> "Q'B, R Row Rotations - Real"/1(x)
  Delay5/1 -> "Q'B, R Row Rotations - Real"/2(y)
  Delay6/1 -> "Q'B, R Row Rotations - Real"/3(u)
  Delay7/1 -> "Q'B, R Row Rotations - Real"/4(v)
  "Q'B, R Row Rotations - Real"/1(x_out) -> Inverse CORDIC Gain4/1(In1)
  "Q'B, R Row Rotations - Real"/3(u_out) -> Inverse CORDIC Gain2/1(In1)
  "Q'B, R Row Rotations - Real"/4(v_out) -> Inverse CORDIC Gain3/1(In1)
  x/1 -> Unit Delay Enabled Synchronous1/1
  u/1 -> Unit Delay Enabled Synchronous/1
  "Q'B, R Row Rotations - Real"/2(y_out) -> Inverse CORDIC Gain1/1(In1)
  Force imaginary part to exactly zero/1(y) -> Real-Imag to Complex/2
  Delay9/1 -> ValidIn to Ready Logic with Delay/3(validIn), Delay10/1
  validIn/1 -> Unit Delay Enabled Synchronous/2, Unit Delay Enabled Synchronous1/2, Delay9/1
  Delay10/1 -> ValidIn to Ready Logic with Delay/2(validIn * z^-1), "Q'B, R Row Rotations - Real"/5(validIn)
  Inverse CORDIC Gain4/1(Out1) -> Real-Imag to Complex/1
  Inverse CORDIC Gain1/1(Out1) -> Force imaginary part to exactly zero/1(u)
  Inverse CORDIC Gain2/1(Out1) -> Real-Imag to Complex1/1
  Inverse CORDIC Gain3/1(Out1) -> Real-Imag to Complex1/2
  "Q'B, R Row Rotations - Real"/5(validOut) -> Unit Delay Enabled Synchronous2/2, Unit Delay Enabled Synchronous3/2, Delay15/1
  Delay15/1 -> validOut/1
  ValidIn to Ready Logic with Delay/1(readyOut) -> ready/1
  "Q'B, R Row Rotations - Real"/6(ready) -> ValidIn to Ready Logic with Delay/1(readyIn)
  Unit Delay Enabled Synchronous/1 -> Complex to Real-Imag1/1
  Unit Delay Enabled Synchronous1/1 -> Complex to Real-Imag/1
  Real-Imag to Complex1/1 -> Unit Delay Enabled Synchronous2/1
  Unit Delay Enabled Synchronous2/1 -> u'/1
  Real-Imag to Complex/1 -> Unit Delay Enabled Synchronous3/1
  Unit Delay Enabled Synchronous3/1 -> x'/1
